simulink model "CryoDetMultiChan_CMB"  (R2016b)
settings: Solver=ode45  StartTime=0.0  StopTime=400e-6  MaxStep=Tclk/4  RelTol=1e-3
values from neighbouring files (symbols this model uses):
  ds_axi = 16    [setupCryoFPGA_CMB.m]
  Fclk = Fadc    (= 307200000)    [setupCryoFPGA_CMB.m]
  lpf = tf(num,den)    [setupCryoFPGA_CMB.m]
  Tclk = 1/Fclk    (= 3.25520833333e-09)    [setupCryoFPGA_CMB.m]
  Ts = 1/Fs    (= 3.25520833333e-09)    [setupADCtoDACloopback.m]    (also in setupCryoFPGA_CMB.m)
undefined symbols (not defined in the file or in its folder): AXI4, i, Lite, xlipgetpartsetting
libraries: xbsIndex_r4 x2215, hdlsllib x6, simulink x3, CryoDetLib x2
(part 3 of 16)

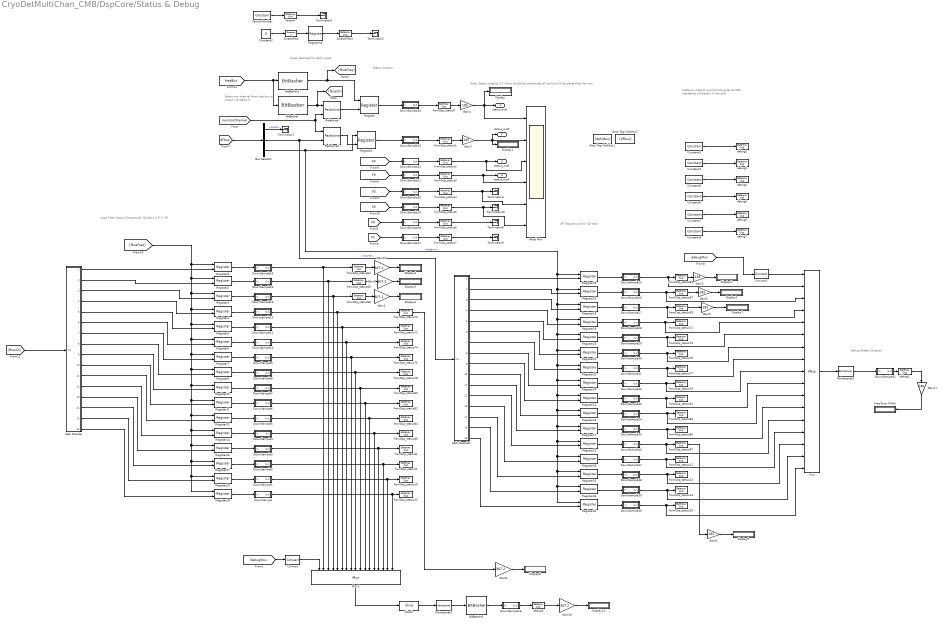
== system CryoDetMultiChan_CMB/DspCore/Status & Debug ==
  note: Loop Filter Output Frequencies (24-bits)
      | = Fi + dF
  note: check latencies for latch inputs
  note: Select one channel from freq bus to output via status 0
  note: Note: Status outputs 2-7 which should be amplitudes all point to F0 as placeholder for now
  note: Status Outputs
  note: Debug Stream Outputs
  note: create an edge to synchronize external DAC interleaver simulation in Simulink
  note: dF Frequency Error (32-bits)
  Addr Decode : Subsystem
  Addr Decode1 : Subsystem
  Ampl Mon : Scope  NumInputPorts=6
  BitBasher : xbsIndex_r4/BitBasher  bitexpr=a={b[28:24]}  display_expr=on  sr_1=a  arith_type1=Unsigned  bin_pt1=0  sr_2=2  arith_type2=Unsigned  bin_pt2=0  sr_3=3  arith_type3=Unsigned  bin_pt3=0  sr_4=4  arith_type4=Unsigned  bin_pt4=0  dbl_ovrd=off  block_type=bitbasher
  BitBasher1 : xbsIndex_r4/BitBasher  bitexpr=a={b[23:0]}  display_expr=on  sr_1=a  arith_type1=Unsigned  bin_pt1=24  sr_2=2  arith_type2=Unsigned  bin_pt2=0  sr_3=3  arith_type3=Unsigned  bin_pt3=0  sr_4=4  arith_type4=Unsigned  bin_pt4=0  dbl_ovrd=off  block_type=bitbasher
  BitBasher3 : xbsIndex_r4/BitBasher  bitexpr=a={8'h00,b[23:0]}  display_expr=off  sr_1=a  arith_type1=Unsigned  bin_pt1=0  sr_2=2  arith_type2=Unsigned  bin_pt2=0  sr_3=3  arith_type3=Unsigned  bin_pt3=0  sr_4=4  arith_type4=Unsigned  bin_pt4=0  dbl_ovrd=off  block_type=bitbasher
  Bus Selector : BusSelector  OutputSignals=Dvalid,channel,freqError
  Constant2 : Constant  Value=0
  Constant3 : xbsIndex_r4/Constant  const=2  gui_display_data_type=Fixed-point  arith_type=Unsigned  n_bits=32  bin_pt=0  preci_type=Single  exp_width=8  frac_width=24  explicit_period=off  period=1  equ=P=C  opselect=C  inp2=PCIN>>17  opr=+  inp1=P  carry=CIN  dbl_ovrd=off  block_type=constant
  Constant4 : xbsIndex_r4/Constant  const=3  gui_display_data_type=Fixed-point  arith_type=Unsigned  n_bits=32  bin_pt=0  preci_type=Single  exp_width=8  frac_width=24  explicit_period=off  period=1  equ=P=C  opselect=C  inp2=PCIN>>17  opr=+  inp1=P  carry=CIN  dbl_ovrd=off  block_type=constant
  Constant5 : xbsIndex_r4/Constant  const=4  gui_display_data_type=Fixed-point  arith_type=Unsigned  n_bits=32  bin_pt=0  preci_type=Single  exp_width=8  frac_width=24  explicit_period=off  period=1  equ=P=C  opselect=C  inp2=PCIN>>17  opr=+  inp1=P  carry=CIN  dbl_ovrd=off  block_type=constant
  Constant6 : xbsIndex_r4/Constant  const=5  gui_display_data_type=Fixed-point  arith_type=Unsigned  n_bits=32  bin_pt=0  preci_type=Single  exp_width=8  frac_width=24  explicit_period=off  period=1  equ=P=C  opselect=C  inp2=PCIN>>17  opr=+  inp1=P  carry=CIN  dbl_ovrd=off  block_type=constant
  Constant7 : xbsIndex_r4/Constant  const=6  gui_display_data_type=Fixed-point  arith_type=Unsigned  n_bits=32  bin_pt=0  preci_type=Single  exp_width=8  frac_width=24  explicit_period=off  period=1  equ=P=C  opselect=C  inp2=PCIN>>17  opr=+  inp1=P  carry=CIN  dbl_ovrd=off  block_type=constant
  Constant8 : xbsIndex_r4/Constant  const=7  gui_display_data_type=Fixed-point  arith_type=Unsigned  n_bits=32  bin_pt=0  preci_type=Single  exp_width=8  frac_width=24  explicit_period=off  period=1  equ=P=C  opselect=C  inp2=PCIN>>17  opr=+  inp1=P  carry=CIN  dbl_ovrd=off  block_type=constant
  Convert : xbsIndex_r4/Convert  gui_display_data_type=Fixed-point  arith_type=Unsigned  n_bits=4  bin_pt=0  float_type=Single  exp_bits=8  fraction_bits=24  quantization=Truncate  overflow=Wrap  en=off  latency=1  pipeline=off  dbl_ovrd=off  block_type=convert
  Convert1 : xbsIndex_r4/Convert  gui_display_data_type=Fixed-point  arith_type=Unsigned  n_bits=4  bin_pt=0  float_type=Single  exp_bits=8  fraction_bits=24  quantization=Truncate  overflow=Wrap  en=off  latency=1  pipeline=off  dbl_ovrd=off  block_type=convert
  Display{,1..10} (11 alike) : Display
      settings: Decimation=144
  DownSample : Subsystem
  DownSample1 : Subsystem
  DownSample10 : Subsystem
  DownSample11 : Subsystem
  DownSample12 : Subsystem
  DownSample13 : Subsystem
  DownSample14 : Subsystem
  DownSample15 : Subsystem
  DownSample16 : Subsystem
  DownSample17 : Subsystem
  DownSample18 : Subsystem
  DownSample19 : Subsystem
  DownSample2 : Subsystem
  DownSample20 : Subsystem
  DownSample21 : Subsystem
  DownSample22 : Subsystem
  DownSample23 : Subsystem
  DownSample24 : Subsystem
  DownSample25 : Subsystem
  DownSample26 : Subsystem
  DownSample27 : Subsystem
  DownSample28 : Subsystem
  DownSample29 : Subsystem
  DownSample3 : Subsystem
  DownSample30 : Subsystem
  DownSample31 : Subsystem
  DownSample32 : Subsystem
  DownSample33 : Subsystem
  DownSample34 : Subsystem
  DownSample35 : Subsystem
  DownSample36 : Subsystem
  DownSample37 : Subsystem
  DownSample38 : Subsystem
  DownSample39 : Subsystem
  DownSample4 : Subsystem
  DownSample40 : Subsystem
  DownSample41 : Subsystem
  DownSample5 : Subsystem
  DownSample6 : Subsystem
  DownSample7 : Subsystem
  DownSample8 : Subsystem
  DownSample9 : Subsystem
  Freq Error (MHz) : Display
      settings: Decimation=144
  Gain{1..2,8,10,12} (5 alike) : Gain  Gain=307.2
  Gain{3..7,9,17} (7 alike) : Gain  Gain=185
  Goto Tag Visibility1 : GotoTagVisibility  GotoTag=dphiBus
  Goto Tag Visibility2 : GotoTagVisibility  GotoTag=dFbus
  Mux : xbsIndex_r4/Mux  inputs=16  en=off  latency=0  precision=Full  arith_type=Unsigned  n_bits=16  bin_pt=14  quantization=Truncate  overflow=Wrap  dbl_ovrd=off  block_type=mux
  Mux1 : xbsIndex_r4/Mux  inputs=16  en=off  latency=0  precision=Full  arith_type=Unsigned  n_bits=16  bin_pt=14  quantization=Truncate  overflow=Wrap  dbl_ovrd=off  block_type=mux
  Register{,1..33} (34 alike) : xbsIndex_r4/Register  init=0  rst=off  en=on  dbl_ovrd=off  block_type=register
  Register34 : xbsIndex_r4/Register  init=0  rst=off  en=off  dbl_ovrd=off  block_type=register
  Reinterpret2 : xbsIndex_r4/Reinterpret  force_arith_type=on  arith_type=Unsigned  force_bin_pt=off  bin_pt=15  block_type=reinterpret
  Reinterpret9 : xbsIndex_r4/Reinterpret  force_arith_type=on  arith_type=Unsigned  force_bin_pt=off  bin_pt=15  block_type=reinterpret
  Relational : xbsIndex_r4/Relational  mode=a=b  op_type=Bool  en=off  latency=0  dbl_ovrd=off  block_type=relational
  Relational1 : xbsIndex_r4/Relational  mode=a=b  op_type=Bool  en=off  latency=0  dbl_ovrd=off  block_type=relational
  ScratchPad : xbsIndex_r4/Gateway In  gui_display_data_type=Fixed-point  arith_type=Unsigned  n_bits=32  bin_pt=0  preci_type=Single  exp_width=8  frac_width=24  rows=1  columns=1  quantization="Round  (unbiased: +/- Inf)"  overflow=Saturate  period=Ts  UseAsADC=off  ADCChannel='1'  interface=AXI4-Lite  automatic_assignment=off  address_offset=hex2dec('F04')  intf_name=''  intf_description=''  default_value=0  timing_constraint=None  locs_specified=off  LOCs={}  io_standard={}  inherit_from_input=off  hdl_port=on  dbl_ovrd=off  block_type=gatewayin
  ScratchPad1 : xbsIndex_r4/Gateway Out  inherit_from_input=on  hdl_port=on  rows=1  columns=1  UseAsDAC=off  DACChannel='1'  interface=AXI4-Lite  automatic_assignment=off  address_offset=hex2dec('F08')  intf_name=''  intf_description=''  timing_constraint=None  locs_specified=off  LOCs={}  io_standard={}  block_type=gatewayout
  Slice2 : xbsIndex_r4/Slice  nbits=24  boolean_output=off  mode=Lower Bit Location + Width  bit1=0  base1=LSB of Input  bit0=0  base0=LSB of Input  dbl_ovrd=off  block_type=slice
  Terminator{1..4,8..10} (7 alike) : Terminator
  Version : xbsIndex_r4/Gateway Out  inherit_from_input=on  hdl_port=on  rows=1  columns=1  UseAsDAC=off  DACChannel='1'  interface=AXI4-Lite  automatic_assignment=off  address_offset=hex2dec('F00')  intf_name=''  intf_description=''  timing_constraint=None  locs_specified=off  LOCs={}  io_standard={}  block_type=gatewayout
  VersionNumber : xbsIndex_r4/Constant  const=hex2dec('00000001')  gui_display_data_type=Fixed-point  arith_type=Unsigned  n_bits=32  bin_pt=0  preci_type=Single  exp_width=8  frac_width=24  explicit_period=off  period=1  equ=P=C  opselect=C  inp2=PCIN>>17  opr=+  inp1=P  carry=CIN  dbl_ovrd=off  block_type=constant
  debug{0..7} (8 alike) : xbsIndex_r4/Gateway Out  inherit_from_input=on  hdl_port=on  rows=1  columns=1  UseAsDAC=off  DACChannel='1'  interface=None  automatic_assignment=on  address_offset=hex2dec('00')  intf_name=''  intf_description=''  timing_constraint=None  locs_specified=off  LOCs={}  io_standard={}  block_type=gatewayout
  fromDsp_status0 : xbsIndex_r4/Gateway Out  inherit_from_input=on  hdl_port=on  rows=1  columns=1  UseAsDAC=off  DACChannel='1'  interface=AXI4-Lite  automatic_assignment=off  address_offset=hex2dec('00')  intf_name=''  intf_description=''  timing_constraint=None  locs_specified=off  LOCs={}  io_standard={}  block_type=gatewayout
  fromDsp_status1 : xbsIndex_r4/Gateway Out  inherit_from_input=on  hdl_port=on  rows=1  columns=1  UseAsDAC=off  DACChannel='1'  interface=AXI4-Lite  automatic_assignment=off  address_offset=hex2dec('04')  intf_name=''  intf_description=''  timing_constraint=None  locs_specified=off  LOCs={}  io_standard={}  block_type=gatewayout
  fromDsp_status10 : xbsIndex_r4/Gateway Out  inherit_from_input=on  hdl_port=on  rows=1  columns=1  UseAsDAC=off  DACChannel='1'  interface=AXI4-Lite  automatic_assignment=off  address_offset=hex2dec('170')  intf_name=''  intf_description=''  timing_constraint=None  locs_specified=off  LOCs={}  io_standard={}  block_type=gatewayout
  fromDsp_status11 : xbsIndex_r4/Gateway Out  inherit_from_input=on  hdl_port=on  rows=1  columns=1  UseAsDAC=off  DACChannel='1'  interface=AXI4-Lite  automatic_assignment=off  address_offset=hex2dec('178')  intf_name=''  intf_description=''  timing_constraint=None  locs_specified=off  LOCs={}  io_standard={}  block_type=gatewayout
  fromDsp_status12 : xbsIndex_r4/Gateway Out  inherit_from_input=on  hdl_port=on  rows=1  columns=1  UseAsDAC=off  DACChannel='1'  interface=AXI4-Lite  automatic_assignment=off  address_offset=hex2dec('164')  intf_name=''  intf_description=''  timing_constraint=None  locs_specified=off  LOCs={}  io_standard={}  block_type=gatewayout
  fromDsp_status13 : xbsIndex_r4/Gateway Out  inherit_from_input=on  hdl_port=on  rows=1  columns=1  UseAsDAC=off  DACChannel='1'  interface=AXI4-Lite  automatic_assignment=off  address_offset=hex2dec('16C')  intf_name=''  intf_description=''  timing_constraint=None  locs_specified=off  LOCs={}  io_standard={}  block_type=gatewayout
  fromDsp_status14 : xbsIndex_r4/Gateway Out  inherit_from_input=on  hdl_port=on  rows=1  columns=1  UseAsDAC=off  DACChannel='1'  interface=AXI4-Lite  automatic_assignment=off  address_offset=hex2dec('174')  intf_name=''  intf_description=''  timing_constraint=None  locs_specified=off  LOCs={}  io_standard={}  block_type=gatewayout
  fromDsp_status15 : xbsIndex_r4/Gateway Out  inherit_from_input=on  hdl_port=on  rows=1  columns=1  UseAsDAC=off  DACChannel='1'  interface=AXI4-Lite  automatic_assignment=off  address_offset=hex2dec('17C')  intf_name=''  intf_description=''  timing_constraint=None  locs_specified=off  LOCs={}  io_standard={}  block_type=gatewayout
  fromDsp_status2 : xbsIndex_r4/Gateway Out  inherit_from_input=on  hdl_port=on  rows=1  columns=1  UseAsDAC=off  DACChannel='1'  interface=AXI4-Lite  automatic_assignment=off  address_offset=hex2dec('08')  intf_name=''  intf_description=''  timing_constraint=None  locs_specified=off  LOCs={}  io_standard={}  block_type=gatewayout
  fromDsp_status3 : xbsIndex_r4/Gateway Out  inherit_from_input=on  hdl_port=on  rows=1  columns=1  UseAsDAC=off  DACChannel='1'  interface=AXI4-Lite  automatic_assignment=off  address_offset=hex2dec('0C')  intf_name=''  intf_description=''  timing_constraint=None  locs_specified=off  LOCs={}  io_standard={}  block_type=gatewayout
  fromDsp_status4 : xbsIndex_r4/Gateway Out  inherit_from_input=on  hdl_port=on  rows=1  columns=1  UseAsDAC=off  DACChannel='1'  interface=AXI4-Lite  automatic_assignment=off  address_offset=hex2dec('10')  intf_name=''  intf_description=''  timing_constraint=None  locs_specified=off  LOCs={}  io_standard={}  block_type=gatewayout
  fromDsp_status5 : xbsIndex_r4/Gateway Out  inherit_from_input=on  hdl_port=on  rows=1  columns=1  UseAsDAC=off  DACChannel='1'  interface=AXI4-Lite  automatic_assignment=off  address_offset=hex2dec('14')  intf_name=''  intf_description=''  timing_constraint=None  locs_specified=off  LOCs={}  io_standard={}  block_type=gatewayout
  fromDsp_status6 : xbsIndex_r4/Gateway Out  inherit_from_input=on  hdl_port=on  rows=1  columns=1  UseAsDAC=off  DACChannel='1'  interface=AXI4-Lite  automatic_assignment=off  address_offset=hex2dec('18')  intf_name=''  intf_description=''  timing_constraint=None  locs_specified=off  LOCs={}  io_standard={}  block_type=gatewayout
  fromDsp_status64 : xbsIndex_r4/Gateway Out  inherit_from_input=on  hdl_port=on  rows=1  columns=1  UseAsDAC=off  DACChannel='1'  interface=AXI4-Lite  automatic_assignment=off  address_offset=hex2dec('100')  intf_name=''  intf_description=''  timing_constraint=None  locs_specified=off  LOCs={}  io_standard={}  block_type=gatewayout
  fromDsp_status65 : xbsIndex_r4/Gateway Out  inherit_from_input=on  hdl_port=on  rows=1  columns=1  UseAsDAC=off  DACChannel='1'  interface=AXI4-Lite  automatic_assignment=off  address_offset=hex2dec('104')  intf_name=''  intf_description=''  timing_constraint=None  locs_specified=off  LOCs={}  io_standard={}  block_type=gatewayout
  fromDsp_status66 : xbsIndex_r4/Gateway Out  inherit_from_input=on  hdl_port=on  rows=1  columns=1  UseAsDAC=off  DACChannel='1'  interface=AXI4-Lite  automatic_assignment=off  address_offset=hex2dec('108')  intf_name=''  intf_description=''  timing_constraint=None  locs_specified=off  LOCs={}  io_standard={}  block_type=gatewayout
  fromDsp_status67 : xbsIndex_r4/Gateway Out  inherit_from_input=on  hdl_port=on  rows=1  columns=1  UseAsDAC=off  DACChannel='1'  interface=AXI4-Lite  automatic_assignment=off  address_offset=hex2dec('10C')  intf_name=''  intf_description=''  timing_constraint=None  locs_specified=off  LOCs={}  io_standard={}  block_type=gatewayout
  fromDsp_status68 : xbsIndex_r4/Gateway Out  inherit_from_input=on  hdl_port=on  rows=1  columns=1  UseAsDAC=off  DACChannel='1'  interface=AXI4-Lite  automatic_assignment=off  address_offset=hex2dec('110')  intf_name=''  intf_description=''  timing_constraint=None  locs_specified=off  LOCs={}  io_standard={}  block_type=gatewayout
  fromDsp_status69 : xbsIndex_r4/Gateway Out  inherit_from_input=on  hdl_port=on  rows=1  columns=1  UseAsDAC=off  DACChannel='1'  interface=AXI4-Lite  automatic_assignment=off  address_offset=hex2dec('114')  intf_name=''  intf_description=''  timing_constraint=None  locs_specified=off  LOCs={}  io_standard={}  block_type=gatewayout
  fromDsp_status7 : xbsIndex_r4/Gateway Out  inherit_from_input=on  hdl_port=on  rows=1  columns=1  UseAsDAC=off  DACChannel='1'  interface=AXI4-Lite  automatic_assignment=off  address_offset=hex2dec('1C')  intf_name=''  intf_description=''  timing_constraint=None  locs_specified=off  LOCs={}  io_standard={}  block_type=gatewayout
  fromDsp_status70 : xbsIndex_r4/Gateway Out  inherit_from_input=on  hdl_port=on  rows=1  columns=1  UseAsDAC=off  DACChannel='1'  interface=AXI4-Lite  automatic_assignment=off  address_offset=hex2dec('118')  intf_name=''  intf_description=''  timing_constraint=None  locs_specified=off  LOCs={}  io_standard={}  block_type=gatewayout
  fromDsp_status71 : xbsIndex_r4/Gateway Out  inherit_from_input=on  hdl_port=on  rows=1  columns=1  UseAsDAC=off  DACChannel='1'  interface=AXI4-Lite  automatic_assignment=off  address_offset=hex2dec('11C')  intf_name=''  intf_description=''  timing_constraint=None  locs_specified=off  LOCs={}  io_standard={}  block_type=gatewayout
  fromDsp_status72 : xbsIndex_r4/Gateway Out  inherit_from_input=on  hdl_port=on  rows=1  columns=1  UseAsDAC=off  DACChannel='1'  interface=AXI4-Lite  automatic_assignment=off  address_offset=hex2dec('120')  intf_name=''  intf_description=''  timing_constraint=None  locs_specified=off  LOCs={}  io_standard={}  block_type=gatewayout
  fromDsp_status73 : xbsIndex_r4/Gateway Out  inherit_from_input=on  hdl_port=on  rows=1  columns=1  UseAsDAC=off  DACChannel='1'  interface=AXI4-Lite  automatic_assignment=off  address_offset=hex2dec('124')  intf_name=''  intf_description=''  timing_constraint=None  locs_specified=off  LOCs={}  io_standard={}  block_type=gatewayout
  fromDsp_status74 : xbsIndex_r4/Gateway Out  inherit_from_input=on  hdl_port=on  rows=1  columns=1  UseAsDAC=off  DACChannel='1'  interface=AXI4-Lite  automatic_assignment=off  address_offset=hex2dec('128')  intf_name=''  intf_description=''  timing_constraint=None  locs_specified=off  LOCs={}  io_standard={}  block_type=gatewayout
  fromDsp_status75 : xbsIndex_r4/Gateway Out  inherit_from_input=on  hdl_port=on  rows=1  columns=1  UseAsDAC=off  DACChannel='1'  interface=AXI4-Lite  automatic_assignment=off  address_offset=hex2dec('12C')  intf_name=''  intf_description=''  timing_constraint=None  locs_specified=off  LOCs={}  io_standard={}  block_type=gatewayout
  fromDsp_status76 : xbsIndex_r4/Gateway Out  inherit_from_input=on  hdl_port=on  rows=1  columns=1  UseAsDAC=off  DACChannel='1'  interface=AXI4-Lite  automatic_assignment=off  address_offset=hex2dec('130')  intf_name=''  intf_description=''  timing_constraint=None  locs_specified=off  LOCs={}  io_standard={}  block_type=gatewayout
  fromDsp_status77 : xbsIndex_r4/Gateway Out  inherit_from_input=on  hdl_port=on  rows=1  columns=1  UseAsDAC=off  DACChannel='1'  interface=AXI4-Lite  automatic_assignment=off  address_offset=hex2dec('134')  intf_name=''  intf_description=''  timing_constraint=None  locs_specified=off  LOCs={}  io_standard={}  block_type=gatewayout
  fromDsp_status78 : xbsIndex_r4/Gateway Out  inherit_from_input=on  hdl_port=on  rows=1  columns=1  UseAsDAC=off  DACChannel='1'  interface=AXI4-Lite  automatic_assignment=off  address_offset=hex2dec('138')  intf_name=''  intf_description=''  timing_constraint=None  locs_specified=off  LOCs={}  io_standard={}  block_type=gatewayout
  fromDsp_status79 : xbsIndex_r4/Gateway Out  inherit_from_input=on  hdl_port=on  rows=1  columns=1  UseAsDAC=off  DACChannel='1'  interface=AXI4-Lite  automatic_assignment=off  address_offset=hex2dec('13C')  intf_name=''  intf_description=''  timing_constraint=None  locs_specified=off  LOCs={}  io_standard={}  block_type=gatewayout
  fromDsp_status8 : xbsIndex_r4/Gateway Out  inherit_from_input=on  hdl_port=on  rows=1  columns=1  UseAsDAC=off  DACChannel='1'  interface=AXI4-Lite  automatic_assignment=off  address_offset=hex2dec('160')  intf_name=''  intf_description=''  timing_constraint=None  locs_specified=off  LOCs={}  io_standard={}  block_type=gatewayout
  fromDsp_status80 : xbsIndex_r4/Gateway Out  inherit_from_input=on  hdl_port=on  rows=1  columns=1  UseAsDAC=off  DACChannel='1'  interface=AXI4-Lite  automatic_assignment=off  address_offset=hex2dec('140')  intf_name=''  intf_description=''  timing_constraint=None  locs_specified=off  LOCs={}  io_standard={}  block_type=gatewayout
  fromDsp_status81 : xbsIndex_r4/Gateway Out  inherit_from_input=on  hdl_port=on  rows=1  columns=1  UseAsDAC=off  DACChannel='1'  interface=AXI4-Lite  automatic_assignment=off  address_offset=hex2dec('144')  intf_name=''  intf_description=''  timing_constraint=None  locs_specified=off  LOCs={}  io_standard={}  block_type=gatewayout
  fromDsp_status82 : xbsIndex_r4/Gateway Out  inherit_from_input=on  hdl_port=on  rows=1  columns=1  UseAsDAC=off  DACChannel='1'  interface=AXI4-Lite  automatic_assignment=off  address_offset=hex2dec('148')  intf_name=''  intf_description=''  timing_constraint=None  locs_specified=off  LOCs={}  io_standard={}  block_type=gatewayout
  fromDsp_status83 : xbsIndex_r4/Gateway Out  inherit_from_input=on  hdl_port=on  rows=1  columns=1  UseAsDAC=off  DACChannel='1'  interface=AXI4-Lite  automatic_assignment=off  address_offset=hex2dec('14C')  intf_name=''  intf_description=''  timing_constraint=None  locs_specified=off  LOCs={}  io_standard={}  block_type=gatewayout
  fromDsp_status84 : xbsIndex_r4/Gateway Out  inherit_from_input=on  hdl_port=on  rows=1  columns=1  UseAsDAC=off  DACChannel='1'  interface=AXI4-Lite  automatic_assignment=off  address_offset=hex2dec('150')  intf_name=''  intf_description=''  timing_constraint=None  locs_specified=off  LOCs={}  io_standard={}  block_type=gatewayout
  fromDsp_status85 : xbsIndex_r4/Gateway Out  inherit_from_input=on  hdl_port=on  rows=1  columns=1  UseAsDAC=off  DACChannel='1'  interface=AXI4-Lite  automatic_assignment=off  address_offset=hex2dec('154')  intf_name=''  intf_description=''  timing_constraint=None  locs_specified=off  LOCs={}  io_standard={}  block_type=gatewayout
  fromDsp_status86 : xbsIndex_r4/Gateway Out  inherit_from_input=on  hdl_port=on  rows=1  columns=1  UseAsDAC=off  DACChannel='1'  interface=AXI4-Lite  automatic_assignment=off  address_offset=hex2dec('158')  intf_name=''  intf_description=''  timing_constraint=None  locs_specified=off  LOCs={}  io_standard={}  block_type=gatewayout
  fromDsp_status87 : xbsIndex_r4/Gateway Out  inherit_from_input=on  hdl_port=on  rows=1  columns=1  UseAsDAC=off  DACChannel='1'  interface=AXI4-Lite  automatic_assignment=off  address_offset=hex2dec('15C')  intf_name=''  intf_description=''  timing_constraint=None  locs_specified=off  LOCs={}  io_standard={}  block_type=gatewayout
  fromDsp_status9 : xbsIndex_r4/Gateway Out  inherit_from_input=on  hdl_port=on  rows=1  columns=1  UseAsDAC=off  DACChannel='1'  interface=AXI4-Lite  automatic_assignment=off  address_offset=hex2dec('168')  intf_name=''  intf_description=''  timing_constraint=None  locs_specified=off  LOCs={}  io_standard={}  block_type=gatewayout
  status_out1 : Outport
  status_out2 : Outport  Port=2
  status_out3 : Outport  Port=3
  status_out4 : Outport  Port=4
  wires:
  fromDsp_status0/1 -> Gain4/1
  fromDsp_status1/1 -> Gain7/1
  fromDsp_status2/1 -> status_out3/1, Ampl Mon/3
  fromDsp_status3/1 -> status_out4/1, Ampl Mon/4
  fromDsp_status7/1 -> Terminator9/1
  fromDsp_status6/1 -> Terminator8/1
  [F0] -> DownSample18/1(In)
  fromDsp_status5/1 -> Ampl Mon/6, Terminator10/1
  [F1] -> DownSample17/1(In)
  [F0] -> DownSample20/1(In)
  DownSample23/1(Out) -> fromDsp_status1/1
  [F0] -> DownSample21/1(In)
  [F0] -> DownSample22/1(In)
  fromDsp_status4/1 -> Ampl Mon/5, Terminator4/1
  [F0] -> DownSample19/1(In)
  [freqBus] -> BitBasher/1, BitBasher1/1
  [monitorChannel] -> Relational1/1, Relational/2
  Relational/1 -> Register/2
  BitBasher1/1 -> [fbusFreq], Register/1
  BitBasher/1 -> [fbusCh], Relational/1
  DownSample24/1(Out) -> fromDsp_status0/1
  [dFbus] -> Bus Selector/1
  Bus Selector/2 -> Addr Decode1/1(In1), Relational1/2  "<channel>"
  Bus Selector/3 -> Register25/1, Register15/1, Register30/1, Register31/1, Register33/1, Register32/1, Register17/1, Register13/1, Register12/1, Register24/1, Register23/1, Register22/1, Register20/1, Register19/1, Register18/1, Register16/1, Register1/1  "<freqError>"
  Relational1/1 -> Register1/2
  Register25/1 -> DownSample25/1(In)
  Register16/1 -> DownSample26/1(In)
  Register18/1 -> DownSample27/1(In)
  Register19/1 -> DownSample28/1(In)
  Register20/1 -> DownSample29/1(In)
  Register22/1 -> DownSample30/1(In)
  Register23/1 -> DownSample31/1(In)
  Register24/1 -> DownSample32/1(In)
  Register12/1 -> DownSample33/1(In)
  Register13/1 -> DownSample34/1(In)
  Register17/1 -> DownSample35/1(In)
  Register15/1 -> DownSample36/1(In)
  [fbusCh] -> Addr Decode/1(In1)
  Addr Decode/1(Out1) -> Register9/2
  Addr Decode/2(Out2) -> Register2/2
  Addr Decode/3(Out3) -> Register3/2
  Addr Decode/4(Out4) -> Register4/2
  Addr Decode/5(Out5) -> Register5/2
  Addr Decode/6(Out6) -> Register6/2
  Addr Decode/7(Out7) -> Register7/2
  Addr Decode/8(Out8) -> Register8/2
  Addr Decode/9(Out9) -> Register10/2
  Addr Decode/10(Out10) -> Register11/2
  Addr Decode/11(Out11) -> Register21/2
  Addr Decode/12(Out12) -> Register14/2
  DownSample4/1(Out) -> fromDsp_status86/1, Mux1/13
  DownSample5/1(Out) -> fromDsp_status84/1, Mux1/12
  DownSample6/1(Out) -> fromDsp_status82/1, Mux1/11
  DownSample7/1(Out) -> fromDsp_status80/1, Mux1/10
  DownSample8/1(Out) -> fromDsp_status78/1, Mux1/9
  DownSample9/1(Out) -> fromDsp_status76/1, Mux1/8
  DownSample10/1(Out) -> fromDsp_status74/1, Mux1/7
  DownSample11/1(Out) -> fromDsp_status72/1, Mux1/6
  DownSample12/1(Out) -> fromDsp_status70/1, Mux1/5
  DownSample13/1(Out) -> fromDsp_status68/1, Mux1/4
  DownSample14/1(Out) -> fromDsp_status66/1, Mux1/3
  [fbusFreq] -> Register9/1, Register2/1, Register4/1, Register5/1, Register6/1, Register7/1, Register8/1, Register10/1, Register11/1, Register21/1, Register26/1, Register27/1, Register29/1, Register28/1, Register14/1, Register3/1
  Addr Decode1/1(Out1) -> Register25/2
  Addr Decode1/2(Out2) -> Register16/2
  Addr Decode1/3(Out3) -> Register18/2
  Addr Decode1/4(Out4) -> Register19/2
  Addr Decode1/5(Out5) -> Register20/2
  Addr Decode1/6(Out6) -> Register22/2
  Addr Decode1/7(Out7) -> Register23/2
  Addr Decode1/8(Out8) -> Register24/2
  Addr Decode1/9(Out9) -> Register12/2
  Addr Decode1/10(Out10) -> Register13/2
  Addr Decode1/11(Out11) -> Register17/2
  Addr Decode1/12(Out12) -> Register15/2
  [debugMux] -> Convert1/1
  [debugMux] -> Convert/1
  DownSample15/1(Out) -> fromDsp_status64/1, Mux1/2
  Slice2/1 -> Reinterpret2/1
  Mux1/1 -> Slice2/1
  Convert1/1 -> Mux/1
  Convert/1 -> Mux1/1
  fromDsp_status65/1 -> Gain3/1
  fromDsp_status67/1 -> Gain6/1
  fromDsp_status64/1 -> Gain12/1
  fromDsp_status66/1 -> Gain1/1
  Gain12/1 -> Display4/1
  Gain1/1 -> Display5/1
  fromDsp_status68/1 -> Gain2/1
  Gain2/1 -> Display6/1
  Gain3/1 -> Display2/1
  Gain6/1 -> Display3/1
  fromDsp_status69/1 -> Gain5/1
  Gain5/1 -> Display7/1
  Gain4/1 -> Ampl Mon/1, Display/1, status_out1/1
  Gain7/1 -> Display1/1, status_out2/1, Ampl Mon/2
  Gain8/1 -> Display8/1
  fromDsp_status70/1 -> Gain8/1
  Gain9/1 -> Display9/1
  fromDsp_status87/1 -> Gain9/1
  Gain10/1 -> Display10/1
  debug0/1 -> Gain10/1
  Addr Decode/13(Out13) -> Register26/2
  Addr Decode/14(Out14) -> Register27/2
  Addr Decode/15(Out15) -> Register29/2
  Addr Decode/16(Out16) -> Register28/2
  DownSample3/1(Out) -> fromDsp_status8/1, Mux1/14
  DownSample2/1(Out) -> fromDsp_status9/1, Mux1/15
  DownSample1/1(Out) -> fromDsp_status10/1, Mux1/16
  DownSample/1(Out) -> fromDsp_status11/1, Mux1/17
  Register30/1 -> DownSample37/1(In)
  Register31/1 -> DownSample38/1(In)
  Register33/1 -> DownSample39/1(In)
  Register32/1 -> DownSample40/1(In)
  Addr Decode1/13(Out13) -> Register30/2
  Addr Decode1/14(Out14) -> Register31/2
  Addr Decode1/15(Out15) -> Register33/2
  Addr Decode1/16(Out16) -> Register32/2
  Reinterpret9/1 -> DownSample41/1(In)
  Mux/1 -> Reinterpret9/1
  Gain17/1 -> Freq Error (MHz)/1
  debug1/1 -> Gain17/1
  Bus Selector/1 -> Terminator1/1  "<Dvalid>"
  Constant3/1 -> debug2/1
  Constant4/1 -> debug3/1
  Constant5/1 -> debug4/1
  Constant6/1 -> debug5/1
  Constant7/1 -> debug6/1
  Constant8/1 -> debug7/1
  ScratchPad1/1 -> Terminator2/1
  Version/1 -> Terminator3/1
  VersionNumber/1 -> Version/1
  ScratchPad/1 -> Register34/1
  Register34/1 -> ScratchPad1/1
  Constant2/1 -> ScratchPad/1
  Register28/1 -> DownSample/1(In)
  Register29/1 -> DownSample1/1(In)
  Register27/1 -> DownSample2/1(In)
  Register26/1 -> DownSample3/1(In)
  Register14/1 -> DownSample4/1(In)
  Register21/1 -> DownSample5/1(In)
  Register11/1 -> DownSample6/1(In)
  Register10/1 -> DownSample7/1(In)
  Register8/1 -> DownSample8/1(In)
  Register7/1 -> DownSample9/1(In)
  Register6/1 -> DownSample10/1(In)
  Register5/1 -> DownSample11/1(In)
  Register4/1 -> DownSample12/1(In)
  Register3/1 -> DownSample13/1(In)
  Register2/1 -> DownSample14/1(In)
  Register9/1 -> DownSample15/1(In)
  Reinterpret2/1 -> BitBasher3/1
  BitBasher3/1 -> DownSample16/1(In)
  DownSample16/1(Out) -> debug0/1
  DownSample21/1(Out) -> fromDsp_status3/1
  DownSample20/1(Out) -> fromDsp_status4/1
  DownSample19/1(Out) -> fromDsp_status5/1
  DownSample18/1(Out) -> fromDsp_status6/1
  DownSample17/1(Out) -> fromDsp_status7/1
  DownSample22/1(Out) -> fromDsp_status2/1
  Register1/1 -> DownSample23/1(In)
  Register/1 -> DownSample24/1(In)
  DownSample25/1(Out) -> Mux/2, fromDsp_status65/1
  DownSample26/1(Out) -> Mux/3, fromDsp_status67/1
  DownSample28/1(Out) -> Mux/5, fromDsp_status71/1
  DownSample27/1(Out) -> Mux/4, fromDsp_status69/1
  DownSample29/1(Out) -> Mux/6, fromDsp_status73/1
  DownSample31/1(Out) -> Mux/8, fromDsp_status77/1
  DownSample32/1(Out) -> Mux/9, fromDsp_status79/1
  DownSample30/1(Out) -> Mux/7, fromDsp_status75/1
  DownSample36/1(Out) -> Mux/13, fromDsp_status87/1
  DownSample33/1(Out) -> fromDsp_status81/1, Mux/10
  DownSample35/1(Out) -> fromDsp_status85/1, Mux/12
  DownSample37/1(Out) -> fromDsp_status12/1, Mux/14
  DownSample40/1(Out) -> Mux/17, fromDsp_status15/1
  DownSample39/1(Out) -> Mux/16, fromDsp_status14/1
  DownSample38/1(Out) -> Mux/15, fromDsp_status13/1
  DownSample34/1(Out) -> Mux/11, fromDsp_status83/1
  DownSample41/1(Out) -> debug1/1
